simulink model "ballOnDrySurface"  (R2017b)
settings: Solver=FixedStepDiscrete  StartTime=0.0  StopTime=inf  FixedStep=1/50  RelTol=1e-3  EnableMultiTasking=on
PreLoadFcn:
  | BOD_startup
undefined symbols (not defined in the file or in its folder): Ad, Ad1, Bd, Bd1, Cd, correction, Discrete, H_unrot, K1, K2, Time
libraries: ctrlSharedLib x2, simulink x2, embdlinuxlib x1
settings Model: SimulationMode=external  Creator=Adam  LastModifiedBy=Josef
settings SolverCC: PositivePriorityOrder=on
settings DataIOCC: LoggingToFile=on
settings OptimizationCC: PassReuseOutputArgsThreshold=0  MaxStackSize=64
settings DebuggingCC: ParameterTunabilityLossMsg=error
settings HardwareCC: ProdBitPerPointer=32  ProdBitPerSizeT=32  ProdBitPerPtrDiffT=32  ProdLargestAtomicInteger=Long  ProdLargestAtomicFloat=Double  ProdWordSize=32  ProdHWDeviceType=ARM Compatible->ARM Cortex  UseEmbeddedCoderFeatures=off
settings SFSimCC: MATLABDynamicMemAlloc=off
settings RTWCC: SystemTargetFile=ert.tlc  HardwareBoard=Raspberry Pi  TemplateMakefile=ert_default_tmf  RTWVerbose=off  Toolchain=GNU GCC Raspberry Pi  TargetLang=C++
settings CodeAppCC: ForceParamTrailComments=on  OperatorAnnotations=on  MangleLength=10  StateflowObjectComments=on  MATLABSourceComments=on
settings ERTTargetCC: TargetLangStandard=C++03 (ISO)  ERTCustomFileBanners=off  SupportContinuousTime=on  SupportNonInlinedSFcns=on  RemoveResetFunc=off  SupportVariableSizeSignals=on  ModelStepFunctionPrototypeControlCompliant=off  ExtMode=on  ExtModeMexArgs='147.32.86.184' 0 17725  ERTSrcFileBannerTemplate=codertarget_code_template.cgt  ERTHdrFileBannerTemplate=codertarget_code_template.cgt  ERTDataSrcFileTemplate=codertarget_code_template.cgt  ERTDataHdrFileTemplate=codertarget_code_template.cgt
settings SimscapeCC: SimscapeNormalizeSystem=off

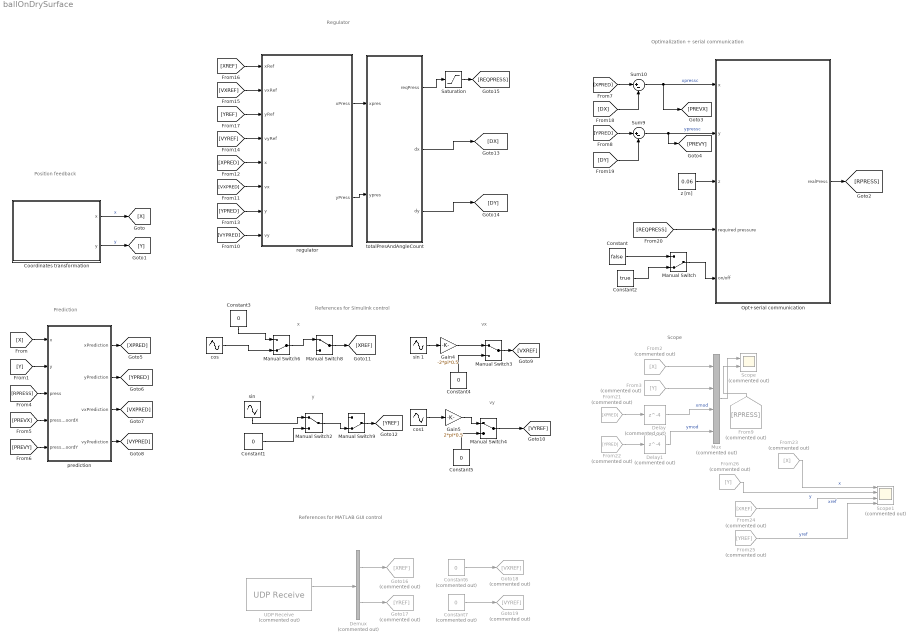
== system ballOnDrySurface ==
  note: vy
  note: y
  note: x
  note: Scope
  note: Optimalization + serial communication
  note: Regulator
  note: References for Simulink control
  note: Prediction
  note: Position feedback
  note: vx
  note: References for MATLAB GUI control
  Constant : Constant  Value=false
  Constant{1,3..5} (4 alike) : Constant  Value=0
  Constant2 : Constant  Value=true
  Constant6 : Constant  Commented=on  Value=0
  Constant7 : Constant  Commented=on  Value=0
  Coordinates transformation : Subsystem
  Delay : Delay  Commented=on  DelayLength=4
  Delay1 : Delay  Commented=on  DelayLength=4
  Demux : Demux  Commented=on  Outputs=2
  From2 : From  Commented=on  GotoTag=X
  From21 : From  Commented=on  GotoTag=XPRED
  From22 : From  Commented=on  GotoTag=YPRED
  From23 : From  Commented=on  GotoTag=X
  From24 : From  Commented=on  GotoTag=XREF
  From25 : From  Commented=on  GotoTag=YREF
  From26 : From  Commented=on  GotoTag=Y
  From3 : From  Commented=on  GotoTag=Y
  From9 : From  Commented=on  GotoTag=RPRESS
  Gain4 : Gain  Gain=-2*pi*0.5
  Gain5 : Gain  Gain=2*pi*0.5
  Goto16 : Goto  Commented=on  GotoTag=XREF
  Goto17 : Goto  Commented=on  GotoTag=YREF
  Goto18 : Goto  Commented=on  GotoTag=VXREF
  Goto19 : Goto  Commented=on  GotoTag=VYREF
  Manual Switch : ManualSwitch  CurrentSetting=0
  Manual Switch{2..4,8} (4 alike) : ManualSwitch
  Manual Switch6 : ManualSwitch  CurrentSetting=0
  Manual Switch9 : ManualSwitch  CurrentSetting=0
  Mux : Mux  Commented=on
  "Opt+serial communication " : Subsystem
  Saturation : Saturate  UpperLimit=3300  LowerLimit=0
  Scope : Scope  Commented=on  NumInputPorts=2
  Scope1 : Scope  Commented=on  NumInputPorts=4
  Sum10 : Sum  Inputs=|+-
  Sum9 : Sum  Inputs=|+-
  UDP Receive : embdlinuxlib/UDP Receive  Commented=on  localURL='0.0.0.0'  localPort=25000  remoteURL='0.0.0.0'  remotePort=-1  recvBufferSize=8192  signalDatatype=double  dims=2  isVarSize=off  showBlockingTime=off  blockingTime=0  sampletime=1/50  blockPlatform=Raspberry Pi
      settings: SourceProductName=Simulink Support Package for Raspberry Pi Hardware  SourceProductBaseCode=RASPPI
  cos : Sin  Amplitude=0.006  Frequency=2*pi*0.5  Phase=pi/2
  cos1 : Sin  Amplitude=0.006  Frequency=2*pi*0.5  Phase=pi/2
  prediction : Subsystem
  "regulator " : Subsystem
  "sin " : Sin  Amplitude=0.006  Frequency=2*pi*0.5
  sin 1 : Sin  Amplitude=0.006  Frequency=2*pi*0.5
  totalPresAndAngleCount : MATLAB Function  TreatAsAtomicUnit=on
  z [m] : Constant  Value=0.06
  wires:
  Delay/1 -> Mux/3  "xmod"
  Delay1/1 -> Mux/4  "ymod"
  Constant/1 -> Manual Switch/1
  Manual Switch/1 -> "Opt+serial communication "/5(on/off)
  z [m]/1 -> "Opt+serial communication "/3(z)
  Constant2/1 -> Manual Switch/2
  Mux/1 -> Scope/1
  Sum10/1 -> [PREVX], "Opt+serial communication "/1(x)  "xpressc"
  totalPresAndAngleCount/1(reqPress) -> Saturation/1
  Coordinates transformation/1(x) -> [X]  "x"
  [X] -> prediction/1(x)
  Coordinates transformation/2(y) -> [Y]  "y"
  [Y] -> prediction/2(y)
  From3/1 -> Mux/2
  From2/1 -> Mux/1
  [RPRESS] -> prediction/3("press ")
  [PREVX] -> prediction/4(pressCoordX)
  [PREVY] -> prediction/5("pressCoordY ")
  prediction/1(xPrediction) -> [XPRED]
  prediction/2(yPrediction) -> [YPRED]
  prediction/3("vxPrediction ") -> [VXPRED]
  prediction/4(vyPrediction) -> [VYPRED]
  [XPRED] -> Sum10/1
  [YPRED] -> Sum9/1
  "Opt+serial communication "/1("realPress ") -> [RPRESS]
  From9/1 -> Scope/2
  [VYPRED] -> "regulator "/8(vy)
  [XPRED] -> "regulator "/5(x)
  Constant4/1 -> Manual Switch3/2
  Constant5/1 -> Manual Switch4/2
  [VYREF] -> "regulator "/4(vyRef)
  Manual Switch3/1 -> [VXREF]
  Manual Switch4/1 -> [VYREF]
  [VXREF] -> "regulator "/2(vxRef)
  Gain4/1 -> Manual Switch3/1
  sin 1/1 -> Gain4/1
  cos1/1 -> Gain5/1
  Gain5/1 -> Manual Switch4/1
  [XREF] -> "regulator "/1(xRef)
  [YREF] -> "regulator "/3(yRef)
  "regulator "/1(xPress) -> totalPresAndAngleCount/1(xpres)
  "regulator "/2(yPress) -> totalPresAndAngleCount/2(ypres)
  totalPresAndAngleCount/2(dx) -> [DX]
  totalPresAndAngleCount/3(dy) -> [DY]
  Saturation/1 -> [REQPRESS]
  Sum9/1 -> [PREVY], "Opt+serial communication "/2(y)  "ypressc"
  [DX] -> Sum10/2
  [DY] -> Sum9/2
  [REQPRESS] -> "Opt+serial communication "/4(required pressure)
  From21/1 -> Delay/1
  From22/1 -> Delay1/1
  [YPRED] -> "regulator "/7(y)
  [VXPRED] -> "regulator "/6(vx)
  "sin "/1 -> Manual Switch2/1
  Constant1/1 -> Manual Switch2/2
  cos/1 -> Manual Switch6/2
  Constant3/1 -> Manual Switch6/1
  From24/1 -> Scope1/3  "xref"
  From23/1 -> Scope1/1  "x"
  From26/1 -> Scope1/2  "y"
  From25/1 -> Scope1/4  "yref"
  Manual Switch8/1 -> [XREF]
  Manual Switch6/1 -> Manual Switch8/1
  Manual Switch9/1 -> [YREF]
  Manual Switch2/1 -> Manual Switch9/2
  Constant6/1 -> Goto18/1
  Constant7/1 -> Goto19/1
  Demux/1 -> Goto16/1
  Demux/2 -> Goto17/1
  UDP Receive/1 -> Demux/1

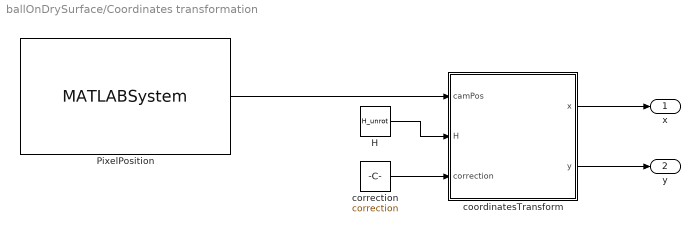
== system ballOnDrySurface/Coordinates transformation ==
  H : Constant  Value=H_unrot
  PixelPosition : MATLABSystem  System=RaspiBallPos  shm_key=3145914  framerate=50  N=1000  objects=1  km=eye( 3 )  notfound=240  execScript=off  concatenateOutputs=off  rotation=off  found_output=off
      mask Type: RaspiBallPos
      mask Display:
      | disp('RaspiBallPos');
      | port_label('output',1,'Position 1 [x;y]');
  coordinatesTransform : MATLAB Function  TreatAsAtomicUnit=on
  correction : Constant  Value=correction
  x : Outport
  y : Outport  Port=2
  wires:
  correction/1 -> coordinatesTransform/3(correction)
  PixelPosition/1 -> coordinatesTransform/1(camPos)
  coordinatesTransform/1(x) -> x/1
  H/1 -> coordinatesTransform/2(H)
  coordinatesTransform/2(y) -> y/1

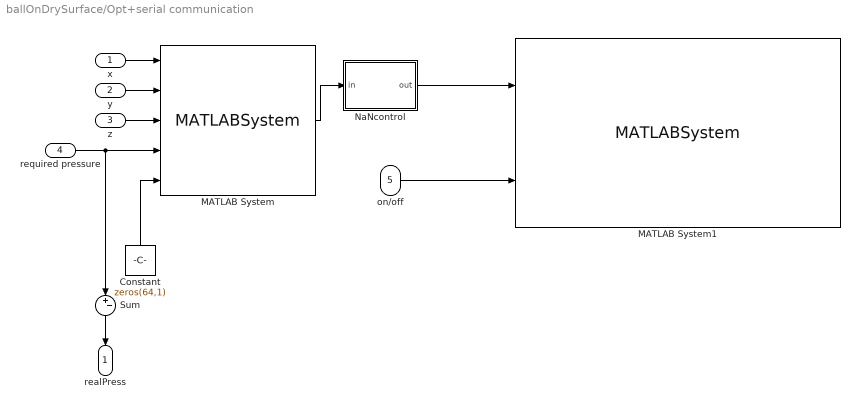
== system ballOnDrySurface/Opt+serial communication  ==
  x : Inport
  y : Inport  Port=2
  z : Inport  Port=3
  required pressure : Inport  Port=4
  on/off : Inport  Port=5
  Constant : Constant  Value=zeros(64,1)
  MATLAB System : MATLABSystem  System=PressurePoints
      mask Type: PressurePoints
      mask Display:
      | disp(['Pressure points' char(10) 'optimization']);
      | port_label('input',1,'x');
      | port_label('input',2,'y');
      | port_label('input',3,'z');
      | port_label('input',4,'Required pressure');
      | port_label('input',5,'Initial condition');
      | port_label('output',1,'Phases');
  MATLAB System1 : MATLABSystem  System=NewGenerator  Port=/dev/ttyUSB0  Baud=230400
      mask Type: NewGenerator
      mask Display:
      | disp(['64 phase generator' char(10) ' Port: /dev/ttyUSB0' char(10) ' Baudrate: 230400']);
      | port_label('input',1,'phases');
      | port_label('input',2,'On/Off');
  NaNcontrol : MATLAB Function  TreatAsAtomicUnit=on
  Sum : Sum  Inputs=|+-
  "realPress " : Outport
  wires:
  y/1 -> MATLAB System/2
  x/1 -> MATLAB System/1
  NaNcontrol/1(out) -> MATLAB System1/1
  Constant/1 -> MATLAB System/5
  z/1 -> MATLAB System/3
  MATLAB System/1 -> NaNcontrol/1(in)
  required pressure/1 -> MATLAB System/4, Sum/1
  on/off/1 -> MATLAB System1/2
  Sum/1 -> "realPress "/1
  ? -> Sum/2

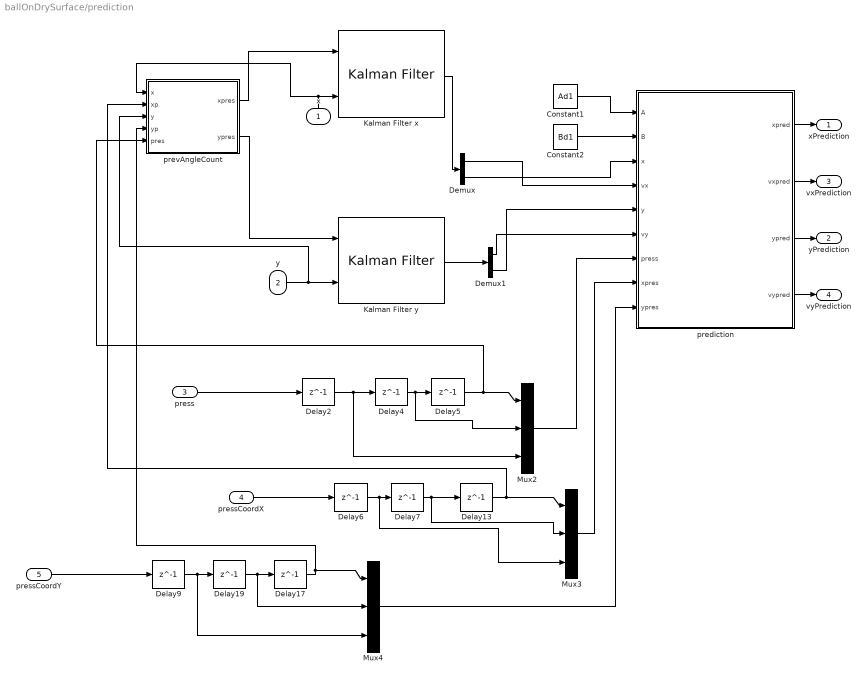
== system ballOnDrySurface/prediction ==
  x : Inport  SampleTime=1/50
  y : Inport  Port=2  SampleTime=1/50
  "press " : Inport  Port=3
  pressCoordX : Inport  Port=4
  "pressCoordY " : Inport  Port=5
  Constant1 : Constant  Value=Ad1  SampleTime=-1
  Constant2 : Constant  Value=Bd1  SampleTime=-1
  Delay{2,4..7,9,13,17,19} (9 alike) : Delay  DelayLength=1
  Demux : Demux  Outputs=2
  Demux1 : Demux  Outputs=2
  Kalman Filter x : ctrlSharedLib/Kalman Filter  TimeDomain=Discrete-Time  UseCurrentEstimator=on  ModelSource=Individual A, B, C, D matrices  ModelSourceVariable=ss(0.95,1,1,0,1)  A=Ad  B=Bd  C=Cd  D=0  NumberOfStates=1  NumberOfInputs=1  NumberOfOutputs=1  InitialEstimateSource=Dialog  X0=[0;0]  P0=10  UseK=off  UseGH=off  NumberOfProcessNoiseInputs=1  G=1  TimeInvariantG=on  H=0  TimeInvariantH=on  Q=[5e-5 0 ; 0 1e-7]  TimeInvariantQ=on  R=7e-12;  TimeInvariantR=on  N=0  TimeInvariantN=on  AddInputPort=on  AddEnablePort=off  OutputEstimatedY=off  OutputP=off  Ts=-1
      settings: SourceProductBaseCode=CT
  Kalman Filter y : ctrlSharedLib/Kalman Filter  TimeDomain=Discrete-Time  UseCurrentEstimator=on  ModelSource=Individual A, B, C, D matrices  ModelSourceVariable=ss(0.95,1,1,0,1)  A=Ad  B=Bd  C=Cd  D=0  NumberOfStates=1  NumberOfInputs=1  NumberOfOutputs=1  InitialEstimateSource=Dialog  X0=[0;0]  P0=10  UseK=off  UseGH=off  NumberOfProcessNoiseInputs=1  G=1  TimeInvariantG=on  H=0  TimeInvariantH=on  Q=[5e-5 0 ; 0 1e-7]  TimeInvariantQ=on  R=7e-12;  TimeInvariantR=on  N=0  TimeInvariantN=on  AddInputPort=on  AddEnablePort=off  OutputEstimatedY=off  OutputP=off  Ts=-1
      settings: SourceProductBaseCode=CT
  Mux2 : Mux  Inputs=3
  Mux3 : Mux  Inputs=3
  Mux4 : Mux  Inputs=3
  prediction : MATLAB Function  TreatAsAtomicUnit=on
  prevAngleCount : MATLAB Function  TreatAsAtomicUnit=on
  xPrediction : Outport
  yPrediction : Outport  Port=2
  "vxPrediction " : Outport  Port=3
  vyPrediction : Outport  Port=4
  wires:
  prediction/1(xpred) -> xPrediction/1
  prediction/3(ypred) -> yPrediction/1
  prediction/2(vxpred) -> "vxPrediction "/1
  prediction/4(vypred) -> vyPrediction/1
  Constant2/1 -> prediction/2(B)
  Constant1/1 -> prediction/1(A)
  x/1 -> prevAngleCount/1(x), Kalman Filter x/2
  y/1 -> prevAngleCount/3(y), Kalman Filter y/2
  Delay4/1 -> Mux2/2, Delay5/1
  Delay5/1 -> prevAngleCount/5(pres), Mux2/1
  Mux2/1 -> prediction/7(press)
  Delay13/1 -> prevAngleCount/2(xp), Mux3/1
  Delay7/1 -> Mux3/2, Delay13/1
  Delay19/1 -> Delay17/1, Mux4/2
  Delay17/1 -> Mux4/1, prevAngleCount/4(yp)
  Mux3/1 -> prediction/8(xpres)
  Mux4/1 -> prediction/9(ypres)
  prevAngleCount/1(xpres) -> Kalman Filter x/1
  Kalman Filter x/1 -> Demux/1
  Demux/1 -> prediction/4(vx)
  prevAngleCount/2(ypres) -> Kalman Filter y/1
  Kalman Filter y/1 -> Demux1/1
  Demux1/1 -> prediction/6(vy)
  Demux/2 -> prediction/3(x)
  Demux1/2 -> prediction/5(y)
  Delay2/1 -> Mux2/3, Delay4/1
  Delay6/1 -> Mux3/3, Delay7/1
  Delay9/1 -> Delay19/1, Mux4/3
  "pressCoordY "/1 -> Delay9/1
  pressCoordX/1 -> Delay6/1
  "press "/1 -> Delay2/1

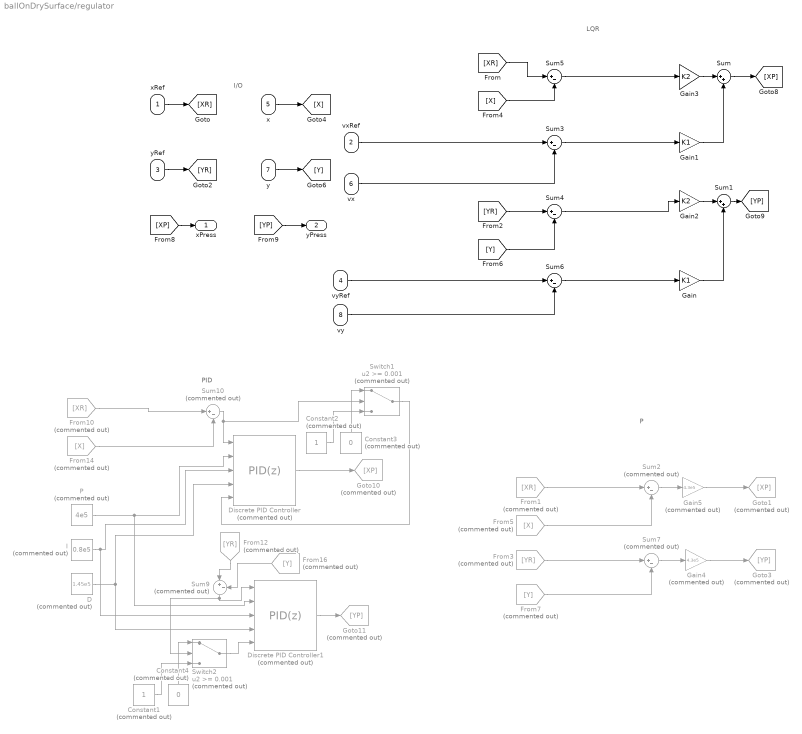
== system ballOnDrySurface/regulator  ==
  note: P
  note: I/O
  note: LQR
  note: PID
  xRef : Inport
  vxRef : Inport  Port=2
  yRef : Inport  Port=3
  vyRef : Inport  Port=4
  x : Inport  Port=5
  vx : Inport  Port=6
  y : Inport  Port=7
  vy : Inport  Port=8
  Constant1 : Constant  Commented=on
  Constant2 : Constant  Commented=on
  Constant3 : Constant  Commented=on  Value=0
  Constant4 : Constant  Commented=on  Value=0
  D : Constant  Commented=on  Value=1.45e5
  Discrete PID Controller : simulink/Continuous/PID Controller  Commented=on  Controller=PID  TimeDomain=Discrete-time  SampleTime=-1  IntegratorMethod=Forward Euler  FilterMethod=Forward Euler  Form=Parallel  UseFilter=off  ControllerParametersSource=external  P=14.5e5  I=0.8e5  D=2e5  N=95.4163407177024  InitialConditionSource=internal  InitialConditionForIntegrator=0  InitialConditionForFilter=0  ExternalReset=rising  LimitOutput=on  UpperSaturationLimit=3300  LowerSaturationLimit=-3300  LinearizeAsGain=off  AntiWindupMode=clamping  Kb=1  TrackingMode=off  Kt=1  PParamMin=[]  PParamMax=[]  IParamMin=[]  IParamMax=[]  DParamMin=[]  DParamMax=[]  NParamMin=[]  NParamMax=[]  KbParamMin=[]  KbParamMax=[]  KtParamMin=[]  KtParamMax=[]  POutMin=[]  POutMax=[]  IOutMin=[]  IOutMax=[]  DOutMin=[]  DOutMax=[]  NOutMin=[]  NOutMax=[]  KbOutMin=[]  KbOutMax=[]  KtOutMin=[]  KtOutMax=[]  IntegratorOutMin=[]  IntegratorOutMax=[]  FilterOutMin=[]  FilterOutMax=[]  SumOutMin=[]  SumOutMax=[]  SumI1OutMin=[]  SumI1OutMax=[]  SumI2OutMin=[]  SumI2OutMax=[]  SumI3OutMin=[]  SumI3OutMax=[]  SumDOutMin=[]  SumDOutMax=[]  SaturationOutMin=[]  SaturationOutMax=[]  IntegratorContinuousStateAttributes=''  IntegratorStateMustResolveToSignalObject=off  IntegratorRTWStateStorageClass=Auto  FilterContinuousStateAttributes=''  FilterStateMustResolveToSignalObject=off  FilterRTWStateStorageClass=Auto  DifferentiatorICPrevScaledInput=0  DifferentiatorOutMin=[]  DifferentiatorOutMax=[]  InitialConditionSetting=State (most efficient)  FilterDiffOutCoefMin=[]  FilterDiffOutCoefMax=[]  SumDenOutMin=[]  SumDenOutMax=[]  SumNumOutMin=[]  SumNumOutMax=[]  ReciprocalOutMin=[]  ReciprocalOutMax=[]  DivideOutMin=[]  DivideOutMax=[]  TunerSelectOption=Transfer Function Based (PID Tuner App)
  Discrete PID Controller1 : simulink/Continuous/PID Controller  Commented=on  Controller=PID  TimeDomain=Discrete-time  SampleTime=-1  IntegratorMethod=Forward Euler  FilterMethod=Forward Euler  Form=Parallel  UseFilter=off  ControllerParametersSource=external  P=14.5e5  I=0.8e5  D=2e5  N=95.4163407177024  InitialConditionSource=internal  InitialConditionForIntegrator=0  InitialConditionForFilter=0  ExternalReset=rising  LimitOutput=on  UpperSaturationLimit=3300  LowerSaturationLimit=-3300  LinearizeAsGain=off  AntiWindupMode=clamping  Kb=1  TrackingMode=off  Kt=1  PParamMin=[]  PParamMax=[]  IParamMin=[]  IParamMax=[]  DParamMin=[]  DParamMax=[]  NParamMin=[]  NParamMax=[]  KbParamMin=[]  KbParamMax=[]  KtParamMin=[]  KtParamMax=[]  POutMin=[]  POutMax=[]  IOutMin=[]  IOutMax=[]  DOutMin=[]  DOutMax=[]  NOutMin=[]  NOutMax=[]  KbOutMin=[]  KbOutMax=[]  KtOutMin=[]  KtOutMax=[]  IntegratorOutMin=[]  IntegratorOutMax=[]  FilterOutMin=[]  FilterOutMax=[]  SumOutMin=[]  SumOutMax=[]  SumI1OutMin=[]  SumI1OutMax=[]  SumI2OutMin=[]  SumI2OutMax=[]  SumI3OutMin=[]  SumI3OutMax=[]  SumDOutMin=[]  SumDOutMax=[]  SaturationOutMin=[]  SaturationOutMax=[]  IntegratorContinuousStateAttributes=''  IntegratorStateMustResolveToSignalObject=off  IntegratorRTWStateStorageClass=Auto  FilterContinuousStateAttributes=''  FilterStateMustResolveToSignalObject=off  FilterRTWStateStorageClass=Auto  DifferentiatorICPrevScaledInput=0  DifferentiatorOutMin=[]  DifferentiatorOutMax=[]  InitialConditionSetting=State (most efficient)  FilterDiffOutCoefMin=[]  FilterDiffOutCoefMax=[]  SumDenOutMin=[]  SumDenOutMax=[]  SumNumOutMin=[]  SumNumOutMax=[]  ReciprocalOutMin=[]  ReciprocalOutMax=[]  DivideOutMin=[]  DivideOutMax=[]  TunerSelectOption=Transfer Function Based (PID Tuner App)
  From1 : From  Commented=on  GotoTag=XR
  From10 : From  Commented=on  GotoTag=XR
  From12 : From  Commented=on  GotoTag=YR
  From14 : From  Commented=on  GotoTag=X
  From16 : From  Commented=on  GotoTag=Y
  From3 : From  Commented=on  GotoTag=YR
  From5 : From  Commented=on  GotoTag=X
  From7 : From  Commented=on  GotoTag=Y
  Gain : Gain  Gain=K1
  Gain1 : Gain  Gain=K1
  Gain2 : Gain  Gain=K2
  Gain3 : Gain  Gain=K2
  Gain4 : Gain  Commented=on  Gain=4.3e5
  Gain5 : Gain  Commented=on  Gain=4.3e5
  Goto1 : Goto  Commented=on  GotoTag=XP
  Goto10 : Goto  Commented=on  GotoTag=XP
  Goto11 : Goto  Commented=on  GotoTag=YP
  Goto3 : Goto  Commented=on  GotoTag=YP
  I : Constant  Commented=on  Value=0.8e5
  P : Constant  Commented=on  Value=4e5
  Sum : Sum  Inputs=|++
  Sum1 : Sum  Inputs=|++
  Sum{2,7,9..10} (4 alike) : Sum  Commented=on  Inputs=|+-
  Sum{3..6} (4 alike) : Sum  Inputs=|+-
  Switch1 : Switch  Commented=on  Threshold=0.001
  Switch2 : Switch  Commented=on  Threshold=0.001
  xPress : Outport
  yPress : Outport  Port=2
  wires:
  Sum3/1 -> Gain1/1
  Sum4/1 -> Gain2/1
  Gain/1 -> Sum1/2
  Sum6/1 -> Gain/1
  Sum5/1 -> Gain3/1
  Gain2/1 -> Sum1/1
  Gain1/1 -> Sum/2
  Gain3/1 -> Sum/1
  xRef/1 -> [XR]
  yRef/1 -> [YR]
  x/1 -> [X]
  y/1 -> [Y]
  [XR] -> Sum5/1
  [YR] -> Sum4/1
  vxRef/1 -> Sum3/1
  vyRef/1 -> Sum6/1
  [X] -> Sum5/2
  vx/1 -> Sum3/2
  [Y] -> Sum4/2
  vy/1 -> Sum6/2
  Sum/1 -> [XP]
  Sum1/1 -> [YP]
  [XP] -> xPress/1
  [YP] -> yPress/1
  Discrete PID Controller/1 -> Goto10/1
  From16/1 -> Sum9/2
  From12/1 -> Sum9/1
  Discrete PID Controller1/1 -> Goto11/1
  From14/1 -> Sum10/2
  From10/1 -> Sum10/1
  Sum10/1 -> Switch1/2, Discrete PID Controller/1
  Sum9/1 -> Switch2/2, Discrete PID Controller1/1
  P/1 -> Discrete PID Controller1/2, Discrete PID Controller/2
  I/1 -> Discrete PID Controller1/3, Discrete PID Controller/3
  D/1 -> Discrete PID Controller1/4, Discrete PID Controller/4
  Gain5/1 -> Goto1/1
  Sum2/1 -> Gain5/1
  Sum7/1 -> Gain4/1
  From7/1 -> Sum7/2
  Gain4/1 -> Goto3/1
  From1/1 -> Sum2/1
  From3/1 -> Sum7/1
  From5/1 -> Sum2/2
  Constant2/1 -> Switch1/3
  Constant3/1 -> Switch1/1
  Constant4/1 -> Switch2/1
  Constant1/1 -> Switch2/3
  Switch2/1 -> Discrete PID Controller1/5
  Switch1/1 -> Discrete PID Controller/5

== matlab function ballOnDrySurface/Opt+serial communication /NaNcontrol ==
  data: in input; out output
function out = NaNcontrol(in)
    if isnan(in)
        out = zeros(64,1);
    else
        out = in;
    end
% % end

== matlab function ballOnDrySurface/Coordinates transformation/coordinatesTransform ==
  data: x output; camPos input; y output; H input; correction input
function [x,y] = coordTrans(camPos, H, correction)
    [x,y] = coordTransform(H, camPos, correction);
end

== matlab function ballOnDrySurface/totalPresAndAngleCount ==
  data: xpres input; ypres input; reqPress output; dx output; dy output
function [reqPress,dx,dy] = totalPresAndAngleCount(xpres,ypres)
reqPress = sqrt(xpres^2+ypres^2);
alpha = atan2(ypres,xpres);
dx = 0.003*cos(alpha);
dy = 0.003*sin(alpha);

== matlab function ballOnDrySurface/prediction/prevAngleCount ==
  data: x input; xpres output; xp input; y input; yp input; pres input; ypres output
function [xpres,ypres] = prevAngleCount(x,xp,y,yp, pres)
angl = atan2((y-yp),(x-xp));
xpres = pres*cos(angl);
ypres = pres*sin(angl);

== matlab function ballOnDrySurface/prediction/prediction ==
  data: A input; B input; x input; vx input; y input; vy input; press input; xpres input; ypres input; xpred output; vxpred output; ypred output; vypred output
function [xpred, vxpred,ypred,vypred] = prediction(A,B,x,vx,y,vy,press,xpres, ypres)

delay = 3;
 ux = zeros(delay,1);
 uy = zeros(delay,1);
 angle = zeros(delay,1);
 angle(1) = atan2(y-ypres(1),x-xpres(1));
 ux(1) = cos(angle(1))*press(1);
 uy(1) = sin(angle(1))*press(1);
 z = [vx;x;vy;y];
for i =1:delay
z = A*z + B*[ux(i);uy(i)];
 if i < delay
 angle(i+1) = atan2(z(4)-ypres(i+1),z(2)-xpres(i+1));
 ux(i+1) = cos(angle(i+1))*press(i+1);
 uy(i+1) = sin(angle(i+1))*press(i+1);
 end
end
 vxpred = z(1);
 xpred = z(2);
 vypred = z(3);
 ypred = z(4);
